simulink model "butterfly_robot_center"  (R2020a)
settings: Solver=VariableStepAuto  StartTime=0.0  StopTime=25  MaxStep=0.01  RelTol=1e-3
undefined symbols (not defined in the file or in its folder): bf
libraries: simulink x5
settings Model: SimulationMode=accelerator  Creator=g-oft  LastModifiedBy=g-oft

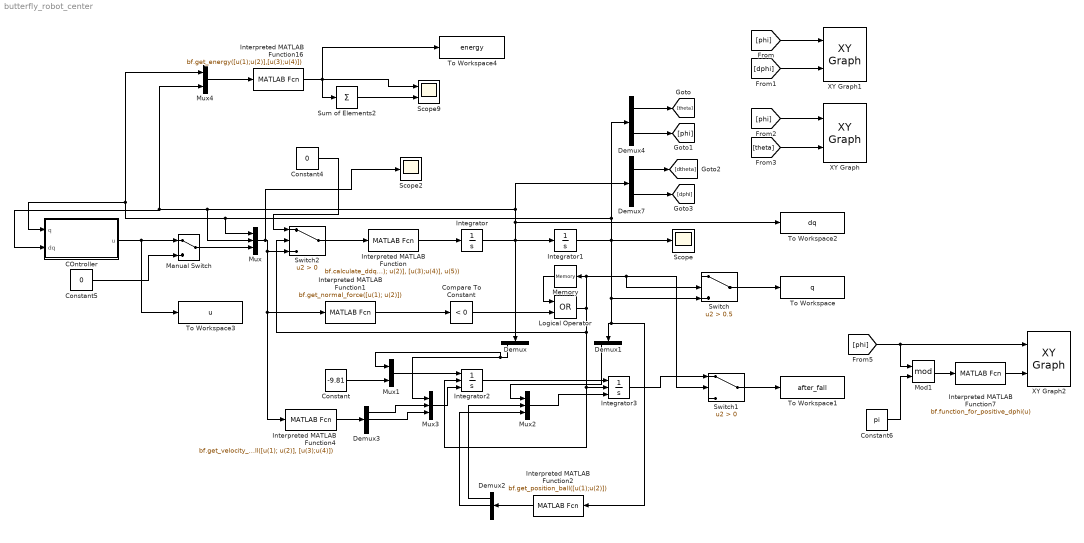
== system butterfly_robot_center ==
  COntroller : Subsystem
  Compare To Constant : simulink/Logic and Bit Operations/Compare To Constant  relop=<  const=0  OutDataTypeStr=boolean
  Constant : Constant  Value=-9.81
  Constant4 : Constant  Value=0
  Constant5 : Constant  Value=0
  Constant6 : Constant  Value=pi
  Demux{,1,4,7} (4 alike) : Demux  Outputs=2
  Demux2 : Demux  Outputs=3
  Demux3 : Demux  Outputs=3
  Integrator : Integrator  InitialCondition=[0;0]
  Integrator1 : Integrator  InitialCondition=[0;0]
  Integrator2 : Integrator  ExternalReset=rising  InitialConditionSource=external
  Integrator3 : Integrator  ExternalReset=rising  InitialConditionSource=external
  Interpreted MATLAB Function : MATLABFcn  MATLABFcn=bf.calculate_ddq([u(1); u(2)], [u(3);u(4)], u(5))
  Interpreted MATLAB Function1 : MATLABFcn  MATLABFcn=bf.get_normal_force([u(1); u(2)])
  Interpreted MATLAB Function16 : MATLABFcn  MATLABFcn=bf.get_energy([u(1);u(2)],[u(3);u(4)])
  Interpreted MATLAB Function2 : MATLABFcn  MATLABFcn=bf.get_position_ball([u(1);u(2)])
  Interpreted MATLAB Function4 : MATLABFcn  MATLABFcn=bf.get_velocity_ball([u(1); u(2)], [u(3);u(4)])
  Interpreted MATLAB Function7 : MATLABFcn  MATLABFcn=bf.function_for_positive_dphi(u)
  Logical Operator : Logic  Operator=OR  AllPortsSameDT=off  OutDataTypeStr=boolean
  Manual Switch : ManualSwitch
  Memory : Memory
  Mod1 : Math  Operator=mod  SaturateOnIntegerOverflow=on
  Mux{,1..3} (4 alike) : Mux  Inputs=3
  Mux4 : Mux  Inputs=2
  Scope : Scope
  Scope2 : Scope
  Scope9 : Scope  NumInputPorts=2
  Sum of Elements2 : Sum  Inputs=+
  Switch : Switch  Criteria=u2 > Threshold  Threshold=0.5
  Switch1 : Switch  Criteria=u2 > Threshold
  Switch2 : Switch  Criteria=u2 > Threshold
  To Workspace : ToWorkspace  VariableName=q  SampleTime=-1
  To Workspace1 : ToWorkspace  VariableName=after_fall  SampleTime=-1
  To Workspace2 : ToWorkspace  VariableName=dq  SampleTime=-1
  To Workspace3 : ToWorkspace  VariableName=u  SampleTime=-1
  To Workspace4 : ToWorkspace  VariableName=energy  SampleTime=-1
  XY Graph : simulink/Sinks/XY Graph  xmin=0  xmax=pi  ymin=-pi  ymax=pi  st=-1
  XY Graph1 : simulink/Sinks/XY Graph  xmin=0  xmax=4  ymin=-1  ymax=5  st=-1
  XY Graph2 : simulink/Sinks/XY Graph  xmin=0  xmax=pi  ymin=-1  ymax=1  st=-1
  wires:
  Constant5/1 -> Manual Switch/2
  COntroller/1(u) -> To Workspace3/1, Manual Switch/1
  Interpreted MATLAB Function16/1 -> Scope9/1, To Workspace4/1, Sum of Elements2/1
  Mux4/1 -> Interpreted MATLAB Function16/1
  [phi] -> XY Graph/1
  Demux7/2 -> [dphi]
  Demux4/1 -> [theta]
  Manual Switch/1 -> Mux/3
  Interpreted MATLAB Function4/1 -> Demux3/1
  Constant4/1 -> Switch2/1
  Switch2/1 -> Interpreted MATLAB Function/1
  Demux4/2 -> [phi]
  Switch1/1 -> To Workspace1/1
  Mux3/1 -> Integrator2/3
  Interpreted MATLAB Function2/1 -> Demux2/1
  Integrator2/1 -> Integrator3/1
  Demux3/2 -> Mux3/3
  Demux2/1 -> Mux2/2
  [phi] -> XY Graph1/1
  Mux1/1 -> Integrator2/1
  Switch/1 -> To Workspace/1
  Sum of Elements2/1 -> Scope9/2
  Memory/1 -> Logical Operator/1
  Demux1/1 -> Mux2/1
  Integrator/1 -> Demux/1, To Workspace2/1, Demux7/1, Mux/2, Mux4/2, COntroller/2(dq), Integrator1/1
  Logical Operator/1 -> Switch2/2, Integrator2/2, Integrator3/2, Memory/1, Switch1/2, Switch/2
  Constant/1 -> Mux1/3
  [dphi] -> XY Graph1/2
  Mux2/1 -> Integrator3/3
  Demux2/2 -> Mux2/3
  Interpreted MATLAB Function1/1 -> Compare To Constant/1
  Compare To Constant/1 -> Logical Operator/2
  Interpreted MATLAB Function7/1 -> XY Graph2/2
  Integrator3/1 -> Switch1/1
  Demux/1 -> Mux1/1, Mux3/1
  Demux7/1 -> [dtheta]
  Integrator1/1 -> Scope/1, Interpreted MATLAB Function2/1, Demux1/1, Switch/3, Mux/1, Mux4/1, COntroller/1(q), Demux4/1
  [phi] -> Mod1/1, XY Graph2/1
  Demux3/1 -> Mux3/2
  Constant6/1 -> Mod1/2
  [theta] -> XY Graph/2
  Mod1/1 -> Interpreted MATLAB Function7/1
  Mux/1 -> Scope2/1, Interpreted MATLAB Function4/1, Interpreted MATLAB Function1/1, Switch2/3
  Interpreted MATLAB Function/1 -> Integrator/1

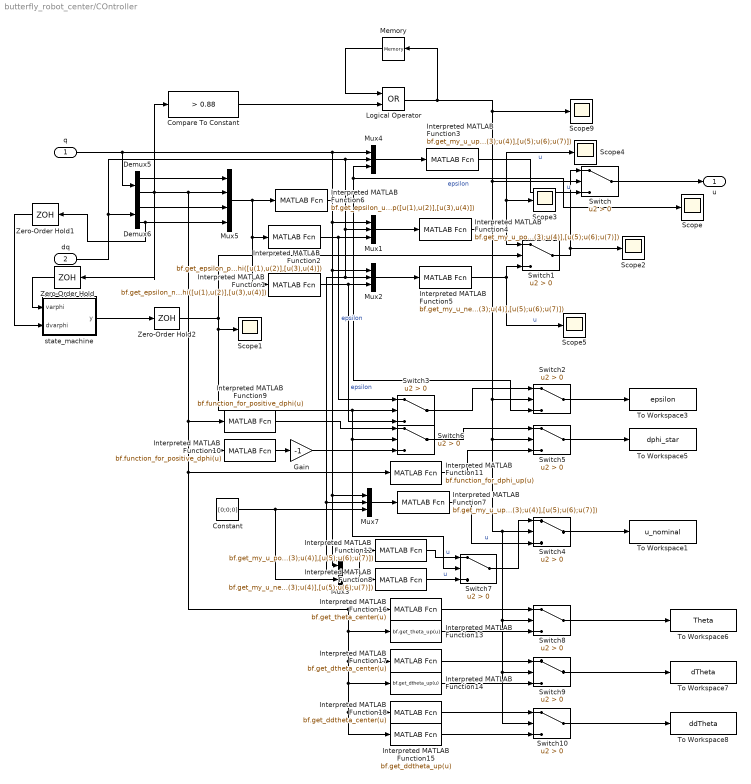
== system butterfly_robot_center/COntroller ==
  q : Inport
  dq : Inport  Port=2
  Compare To Constant : simulink/Logic and Bit Operations/Compare To Constant  relop=>  const=0.88  OutDataTypeStr=boolean
  Constant : Constant  Value=[0;0;0]
  Demux5 : Demux  Outputs=2
  Demux6 : Demux  Outputs=2
  Gain : Gain  Gain=-1
  Interpreted MATLAB Function1 : MATLABFcn  MATLABFcn=bf.get_epsilon_negative_dphi([u(1),u(2)],[u(3),u(4)])
  Interpreted MATLAB Function10 : MATLABFcn  MATLABFcn=bf.function_for_positive_dphi(u)
  Interpreted MATLAB Function11 : MATLABFcn  MATLABFcn=bf.function_for_dphi_up(u)
  Interpreted MATLAB Function12 : MATLABFcn  MATLABFcn=bf.get_my_u_positive_dphi([u(1);u(2)],[u(3);u(4)],[u(5);u(6);u(7)])
  Interpreted MATLAB Function13 : MATLABFcn  MATLABFcn=bf.get_theta_up(u)
  Interpreted MATLAB Function14 : MATLABFcn  MATLABFcn=bf.get_dtheta_up(u)
  Interpreted MATLAB Function15 : MATLABFcn  MATLABFcn=bf.get_ddtheta_up(u)
  Interpreted MATLAB Function16 : MATLABFcn  MATLABFcn=bf.get_theta_center(u)
  Interpreted MATLAB Function17 : MATLABFcn  MATLABFcn=bf.get_dtheta_center(u)
  Interpreted MATLAB Function18 : MATLABFcn  MATLABFcn=bf.get_ddtheta_center(u)
  Interpreted MATLAB Function2 : MATLABFcn  MATLABFcn=bf.get_epsilon_positive_dphi([u(1),u(2)],[u(3),u(4)])
  Interpreted MATLAB Function3 : MATLABFcn  MATLABFcn=bf.get_my_u_up([u(1);u(2)],[u(3);u(4)],[u(5);u(6);u(7)])
  Interpreted MATLAB Function4 : MATLABFcn  MATLABFcn=bf.get_my_u_positive_dphi([u(1);u(2)],[u(3);u(4)],[u(5);u(6);u(7)])
  Interpreted MATLAB Function5 : MATLABFcn  MATLABFcn=bf.get_my_u_negative_dphi([u(1);u(2)],[u(3);u(4)],[u(5);u(6);u(7)])
  Interpreted MATLAB Function6 : MATLABFcn  MATLABFcn=bf.get_epsilon_up([u(1),u(2)],[u(3),u(4)])
  Interpreted MATLAB Function7 : MATLABFcn  MATLABFcn=bf.get_my_u_up([u(1);u(2)],[u(3);u(4)],[u(5);u(6);u(7)])
  Interpreted MATLAB Function8 : MATLABFcn  MATLABFcn=bf.get_my_u_negative_dphi([u(1);u(2)],[u(3);u(4)],[u(5);u(6);u(7)])
  Interpreted MATLAB Function9 : MATLABFcn  MATLABFcn=bf.function_for_positive_dphi(u)
  Logical Operator : Logic  Operator=OR  AllPortsSameDT=off  OutDataTypeStr=boolean
  Memory : Memory
  Mux{1..4,7} (5 alike) : Mux  Inputs=3
  Mux5 : Mux
  Scope : Scope  NumInputPorts=3
  Scope{1..5,9} (6 alike) : Scope
  Switch{,1..10} (11 alike) : Switch  Criteria=u2 > Threshold
  To Workspace1 : ToWorkspace  VariableName=u_nominal  SampleTime=-1
  To Workspace3 : ToWorkspace  VariableName=epsilon  SampleTime=-1
  To Workspace5 : ToWorkspace  VariableName=dphi_star  SampleTime=-1
  To Workspace6 : ToWorkspace  VariableName=Theta  SampleTime=-1
  To Workspace7 : ToWorkspace  VariableName=dTheta  SampleTime=-1
  To Workspace8 : ToWorkspace  VariableName=ddTheta  SampleTime=-1
  Zero-Order Hold : ZeroOrderHold  SampleTime=-1
  Zero-Order Hold1 : ZeroOrderHold  SampleTime=-1
  Zero-Order Hold2 : ZeroOrderHold  SampleTime=-1
  state_machine : MATLAB Function  TreatAsAtomicUnit=on
  u : Outport
  wires:
  q/1 -> Demux5/1, Mux3/1, Mux7/1, Mux2/1, Mux1/1, Mux4/1
  Mux5/1 -> Interpreted MATLAB Function2/1, Interpreted MATLAB Function1/1, Interpreted MATLAB Function6/1
  Demux5/2 -> Interpreted MATLAB Function15/1, Interpreted MATLAB Function18/1, Interpreted MATLAB Function14/1, Interpreted MATLAB Function17/1, Interpreted MATLAB Function13/1, Interpreted MATLAB Function16/1, Interpreted MATLAB Function11/1, Interpreted MATLAB Function10/1, Interpreted MATLAB Function9/1, Mux5/2, Zero-Order Hold/1, Compare To Constant/1
  Demux6/1 -> Mux5/3
  dq/1 -> Mux4/2, Mux3/2, Mux7/2, Mux2/2, Mux1/2, Demux6/1
  Mux4/1 -> Interpreted MATLAB Function3/1
  Demux6/2 -> Zero-Order Hold1/1, Mux5/4
  Interpreted MATLAB Function6/1 -> Scope/2, Mux4/3, Switch2/3  "epsilon"
  Demux5/1 -> Mux5/1
  Memory/1 -> Logical Operator/1
  Mux1/1 -> Interpreted MATLAB Function4/1
  Mux2/1 -> Interpreted MATLAB Function5/1
  Interpreted MATLAB Function4/1 -> Scope3/1, Scope4/1, Switch1/1  "u"
  Interpreted MATLAB Function5/1 -> Switch1/3, Scope5/1  "u"
  Interpreted MATLAB Function3/1 -> Switch/3  "u"
  Switch1/1 -> Switch/1, Scope2/1
  Interpreted MATLAB Function2/1 -> Switch3/1, Mux1/3  "epsilon"
  state_machine/1(y) -> Zero-Order Hold2/1
  Zero-Order Hold/1 -> state_machine/1(varphi)
  Zero-Order Hold1/1 -> state_machine/2(dvarphi)
  Zero-Order Hold2/1 -> Switch7/2, Switch6/2, Switch3/2, Scope1/1, Switch1/2
  Interpreted MATLAB Function1/1 -> Switch3/3, Mux2/3  "epsilon"
  Switch/1 -> u/1
  Compare To Constant/1 -> Logical Operator/2
  Switch3/1 -> Switch2/1
  Switch2/1 -> To Workspace3/1
  Mux3/1 -> Interpreted MATLAB Function12/1, Interpreted MATLAB Function8/1
  Mux7/1 -> Interpreted MATLAB Function7/1
  Constant/1 -> Mux3/3, Mux7/3
  Switch4/1 -> To Workspace1/1
  Logical Operator/1 -> Memory/1, Scope9/1, Switch5/2, Switch10/2, Switch9/2, Switch8/2, Switch4/2, Switch2/2, Switch/2
  Switch6/1 -> Switch5/1
  Switch5/1 -> To Workspace5/1
  Interpreted MATLAB Function9/1 -> Switch6/1
  Interpreted MATLAB Function10/1 -> Gain/1
  Gain/1 -> Switch6/3
  Interpreted MATLAB Function11/1 -> Switch5/3
  Interpreted MATLAB Function8/1 -> Switch7/3  "u"
  Interpreted MATLAB Function12/1 -> Switch7/1  "u"
  Switch7/1 -> Switch4/1
  Interpreted MATLAB Function7/1 -> Switch4/3  "u"
  Interpreted MATLAB Function13/1 -> Switch8/3
  Interpreted MATLAB Function14/1 -> Switch9/3
  Interpreted MATLAB Function15/1 -> Switch10/3
  Interpreted MATLAB Function16/1 -> Switch8/1
  Interpreted MATLAB Function17/1 -> Switch9/1
  Interpreted MATLAB Function18/1 -> Switch10/1
  Switch8/1 -> To Workspace6/1
  Switch9/1 -> To Workspace7/1
  Switch10/1 -> To Workspace8/1

== matlab function butterfly_robot_center/COntroller/state_machine ==
  data: varphi input; y output; dvarphi input
function y = fcn(varphi, dvarphi)
    persistent state 
    if isempty(state)
        state = 1;
    end
    if dvarphi <= 0.01 && varphi > 2
        state = -1; 
    end
    if dvarphi >= -0.01 && varphi < 1.2
        state = 1;
    end
y = state;
